simulink model "dataget_continuous"  (R2022a)
settings: Solver=ode45  StartTime=0.0  StopTime=time  RelTol=1e-8  AbsTol=1e-10
values from neighbouring files (symbols this model uses):
  A0 = [0, 1; -1, -1.4]    [code_tra.m]
  B0 = [0; 1]    [code_tra.m]
  C0 = [1, 0]    [code_tra.m]
  D0 = [0]    [code_tra.m]
  ran_max = 20    [code_tra.m]
  ran_min = 5    [code_tra.m]
  sam_time = 20    [code_tra.m]
  seed = randi(2^31-2)    [code_tra.m]
  Td = 0.001    [code_tra.m]
  Ts_log = 0.001    [code_tra.m]
  wav = 0.7    [code_tra.m]
undefined symbols (not defined in the file or in its folder): AA_s, AT, b0, b1, b2, b3, BB_s, BT, CC_s, CT, DD_s, DT, gamma, omega, rho, sigma, w0, w1, w2, w3
libraries: simulink x1
settings Model: Creator=IDS_PC  LastModifiedBy=IDS_PC
settings SolverCC: SolverResetMethod=Robust
settings DebuggingCC: AlgebraicLoopMsg=none

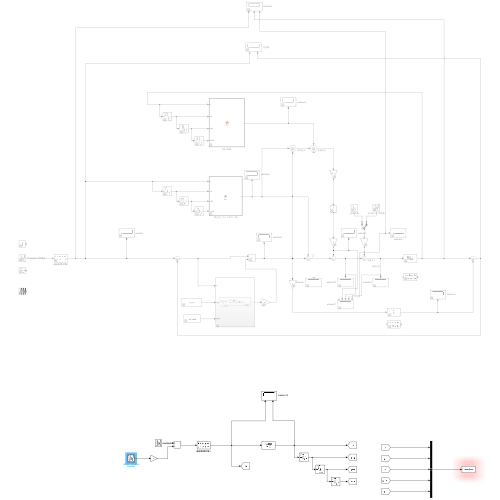
[thumbnail: Simulink's stored preview of the top-level diagram]
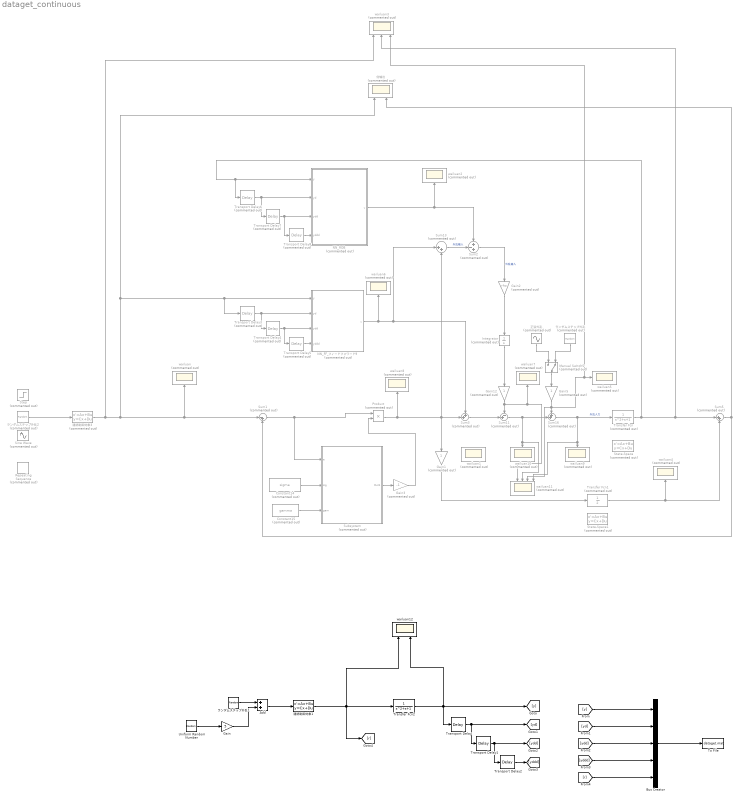
== system dataget_continuous ==
  " 正弦外乱" : Sin  Commented=on  Amplitude=wav  Bias=1  Frequency=omega  Phase=1  SampleTime=0
  Add : Sum
  Bus Creator : BusCreator  Inputs=5
  Constant14 : Constant  Commented=on  Value=sigma  SampleTime=0
  Constant15 : Constant  Commented=on  Value=gamma  SampleTime=0
  Gain : Gain  Gain=5
  Gain1 : Gain  Commented=on
  Gain12 : Gain  Commented=on
  Gain2 : Gain  Commented=on  Gain=rho
  Gain3 : Gain  Commented=on  Gain=-1
  Gain5 : Gain  Commented=on
  Integrator : Integrator  Commented=on
  Manual Switch5 : ManualSwitch  Commented=on  CurrentSetting=0
  NN_FF_フィードフォワード9 : MATLAB Function  Commented=on  TreatAsAtomicUnit=on
  NN_ROB : MATLAB Function  Commented=on  TreatAsAtomicUnit=on
  Product : Product  Commented=on
  Repeating Sequence : simulink/Sources/Repeating Sequence  Commented=on  rep_seq_t=[0 2]  rep_seq_y=[0 2]
  Sine Wave : Sin  Commented=on  SampleTime=0
  State-Space : StateSpace  Commented=on  A=AT  B=BT  C=CT  D=DT  InitialCondition=0
  State-Space1 : StateSpace  Commented=on  A=AA_s  B=BB_s  C=CC_s  D=DD_s  InitialCondition=0
  Step : Step  Commented=on  SampleTime=0
  Subsystem : Subsystem  Commented=on
  Sum1 : Sum  Commented=on  Inputs=|-+
  Sum11 : Sum  Commented=on  Inputs=-+|
  Sum13 : Sum  Commented=on  Inputs=|++
  Sum16 : Sum  Commented=on  Inputs=++|
  Sum2 : Sum  Commented=on  Inputs=+-+
  Sum3 : Sum  Commented=on  Inputs=++|
  Sum5 : Sum  Commented=on  Inputs=|++
  To File : ToFile  Filename=dataget.mat  MatrixName=dataget  SampleTime=Ts_log
  Transfer Fcn : TransferFcn  Commented=on  Denominator=[1 1 1]
  Transfer Fcn1 : TransferFcn  Commented=on  Denominator=[2]
  Transfer Fcn2 : TransferFcn  Denominator=[1 1 1]
  Transport Delay : TransportDelay  DelayTime=Td
  Transport Delay1 : TransportDelay  DelayTime=Td
  Transport Delay2 : TransportDelay  DelayTime=Td
  Transport Delay{3..8} (6 alike) : TransportDelay  Commented=on  DelayTime=Td
  Uniform Random Number : UniformRandomNumber  Minimum=-wav  Maximum=wav  Seed=seed+100  SampleTime=29
  wailuan{,1..2,4..10} (10 alike) : Scope  Commented=on
  wailuan11 : Scope  Commented=on  NumInputPorts=5
  wailuan12 : Scope  NumInputPorts=2
  wailuan3 : Scope  Commented=on  NumInputPorts=3
  ランダムステップ外乱 : UniformRandomNumber  Commented=on  Minimum=-wav  Maximum=wav  Seed=seed+5  SampleTime=32
  ランダムステップ外乱1 : UniformRandomNumber  Minimum=ran_min  Maximum=ran_max  Seed=seed  SampleTime=sam_time
  ランダムステップ外乱2 : UniformRandomNumber  Commented=on  Minimum=-5  Maximum=5  Seed=seed+5  SampleTime=32
  伪输出 : Scope  Commented=on  NumInputPorts=2
  連続制御対象1 : StateSpace  A=A0  B=B0  C=C0  D=D0  InitialCondition=0
  連続制御対象3 : StateSpace  Commented=on  A=A0  B=B0  C=C0  D=D0  InitialCondition=0
  wires:
  Sum16/1 -> Transfer Fcn/1, wailuan11/5, wailuan9/1  "外乱入力"
  Gain5/1 -> wailuan11/4, wailuan3/3, wailuan5/1, Sum16/1
  Manual Switch5/1 -> Gain5/1
  ランダムステップ外乱/1 -> Manual Switch5/2
  " 正弦外乱"/1 -> Manual Switch5/1
  Sum11/1 -> Sum16/2, wailuan11/3, wailuan10/1
  Gain12/1 -> Sum11/1, wailuan11/2, wailuan7/1
  Product/1 -> Gain1/1, Sum3/2, Sum13/2, wailuan8/1
  Transfer Fcn/1 -> wailuan3/2, Sum5/1, Transport Delay6/1, NN_ROB/1(y)
  連続制御対象3/1 -> wailuan3/1, Sum1/1, wailuan/1, 伪输出/1, Transport Delay3/1, NN_FF_フィードフォワード9/1(y)
  NN_FF_フィードフォワード9/1(v) -> Sum3/1, Sum13/1, wailuan6/1
  NN_ROB/1(v) -> Sum2/1, wailuan2/1
  Sum13/1 -> Sum2/2  "外乱输入"
  Gain2/1 -> Integrator/1
  Sum2/1 -> Gain2/1  "外乱输入"
  Integrator/1 -> Gain12/1
  Transport Delay5/1 -> NN_FF_フィードフォワード9/4(yddd)
  Transport Delay4/1 -> Transport Delay5/1, NN_FF_フィードフォワード9/3(ydd)
  Transport Delay3/1 -> Transport Delay4/1, NN_FF_フィードフォワード9/2(yd)
  Transport Delay8/1 -> NN_ROB/4(yddd)
  Transport Delay6/1 -> Transport Delay7/1, NN_ROB/2(yd)
  Transport Delay7/1 -> Transport Delay8/1, NN_ROB/3(ydd)
  Gain1/1 -> Transfer Fcn1/1
  Transfer Fcn1/1 -> Sum5/2, wailuan4/1
  ランダムステップ外乱2/1 -> 連続制御対象3/1
  Sum5/1 -> 伪输出/2, Sum1/2
  Sum1/1 -> Product/1, Subsystem/1(e)
  Constant14/1 -> Subsystem/2(sig)
  Constant15/1 -> Subsystem/3(gam)
  Subsystem/1(Out1) -> Gain3/1
  Gain3/1 -> Product/2
  Sum3/1 -> Sum11/2
  Bus Creator/1 -> To File/1
  連続制御対象1/1 -> Transfer Fcn2/1, wailuan12/1, [r]
  Transfer Fcn2/1 -> wailuan12/2, Transport Delay/1, [y]
  Add/1 -> 連続制御対象1/1
  Transport Delay/1 -> [yd], Transport Delay1/1
  Transport Delay1/1 -> Transport Delay2/1, [ydd]
  Transport Delay2/1 -> [yddd]
  [y] -> Bus Creator/1
  [yd] -> Bus Creator/2
  [ydd] -> Bus Creator/3
  [yddd] -> Bus Creator/4
  [r] -> Bus Creator/5
  ランダムステップ外乱1/1 -> Add/1
  Uniform Random Number/1 -> Gain/1
  Gain/1 -> Add/2

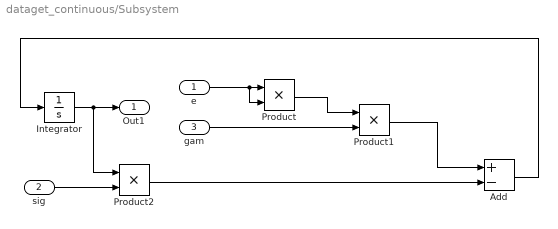
== system dataget_continuous/Subsystem ==
  e : Inport
  sig : Inport  Port=2
  gam : Inport  Port=3
  Add : Sum  Inputs=+-
  Integrator : Integrator  UpperSaturationLimit=999999999999999999  LowerSaturationLimit=-9999999999999999
  Product : Product
  Product1 : Product
  Product2 : Product
  Out1 : Outport
  wires:
  e/1 -> Product/2, Product/1
  Product/1 -> Product1/1
  gam/1 -> Product1/2
  Integrator/1 -> Product2/1, Out1/1
  sig/1 -> Product2/2
  Product2/1 -> Add/2
  Product1/1 -> Add/1
  Add/1 -> Integrator/1

== matlab function dataget_continuous/NN_ROB ==
  data: y input; yd input; ydd input; yddd input; v output; w0 parameter; w1 parameter; w2 parameter; w3 parameter; b0 parameter; b1 parameter; b2 parameter; b3 parameter
function v = fcn(y, yd, ydd, yddd, w0, w1, w2, w3, b0, b1, b2, b3)

    x = [yddd, ydd, yd, y];
    x = x.';

    s1= (transpose(w0)) * x + b0;
    x1= max(0,s1);     %relu 
    s2= (transpose(w1)) * x1 + b1;
    x2= max(0,s2);     %relu
    s3= (transpose(w2)) * x2 + b2;
    x3= max(0,s3);     %relu
    s4= (transpose(w3)) * x3 + b3;

v=s4;

== matlab function dataget_continuous/NN_FF_フィードフォワード9 ==
  data: y input; yd input; ydd input; yddd input; v output; w0 parameter; w1 parameter; w2 parameter; w3 parameter; b0 parameter; b1 parameter; b2 parameter; b3 parameter
function v = fcn(y, yd, ydd, yddd, w0, w1, w2, w3, b0, b1, b2, b3)

    x = [yddd, ydd, yd, y];
    x = x.';

    s1= (transpose(w0)) * x + b0;
    x1= max(0,s1);     %relu 
    s2= (transpose(w1)) * x1 + b1;
    x2= max(0,s2);     %relu
    s3= (transpose(w2)) * x2 + b2;
    x3= max(0,s3);     %relu
    s4= (transpose(w3)) * x3 + b3;

v=s4;
